simulink model "AFE_3L_DCP_DCN"  (R2013a)
settings: Solver=FixedStepDiscrete  SolverMode=SingleTasking  StartTime=0.0  StopTime=inf  FixedStep=Tpas  RelTol=1e-3
values from neighbouring files (symbols this model uses):
  Cbus = 300e-3    (= 0.3)    [AFE_FV_Params.m]
  fmod4Q = 1e3    (= 1000)    [AFE_FV_Params.m]
  Freq = 50    [AFE_FV_Params.m]
  IC = 2    [AFE_FV_Params.m]
  IDCP = (PDCP+Numd(2)/Dend(1))/Ts    [AFE_FV_Params.m]
  Iv = (Pv+Numdv(2)/Dendv(1))/Tsv    [AFE_FV_Params.m]
  Kac = 1/(Vac*sqrt(2/3))    [AFE_FV_Params.m]
  L = .1    (= 0.1)    [AFE_FV_Params.m]
  Lac = 8.1487e-04    (= 0.00081487)    [AFE_FV_Params.m]
  Lcoup = 10e-6    (= 1e-05)    [AFE_FV_Params.m]
  PC = 0.001    [AFE_FV_Params.m]
  PDCP = Numd(1)/Dend(1)    [AFE_FV_Params.m]
  Pv = Numdv(1)/Dendv(1)    [AFE_FV_Params.m]
  R = .28    (= 0.28)    [AFE_FV_Params.m]
  Satv = 1000    [AFE_FV_Params.m]
  Tpas = 1e-6    (= 1e-06)    [AFE_FV_Params.m]
  Vac = 2000    [AFE_FV_Params.m]
  Vdc = 5000    [AFE_FV_Params.m]
undefined symbols (not defined in the file or in its folder): KLPDCP, Rac, TLPDCP
libraries: powerlib x78, simulink x46, powerlib_meascontrol x16
settings Model: Creator=LiberT  LastModifiedBy=Francis
settings DataIOCC: SignalLoggingSaveFormat=ModelDataLogs
settings OptimizationCC: ExpressionDepthLimit=2147483647
settings DebuggingCC: MultiTaskDSMMsg=warning  MultiTaskCondExecSysMsg=none  FcnCallInpInsideContextMsg=EnableAllAsWarning  StrictBusMsg=None
settings RTWCC: IncludeERTFirstTime=on

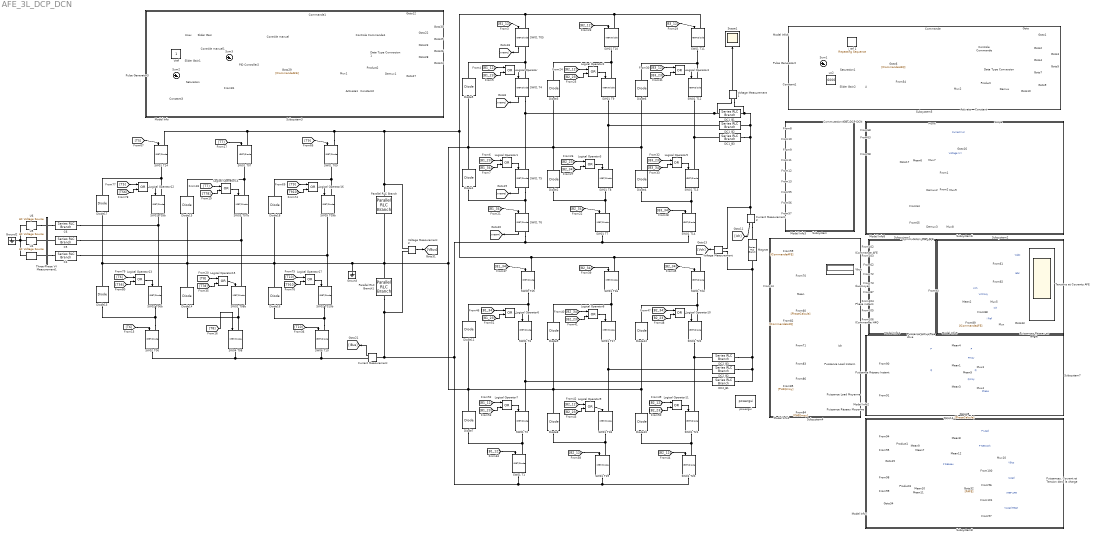
== system AFE_3L_DCP_DCN ==
  " " : ManualSwitch
  " 4" : ManualSwitch  CurrentSetting=0
  Activate : Constant  Value=0
  Activate1 : Constant  Value=0
  C4 : powerlib/Elements/Series RLC Branch  LConnTagsString=__new0  RConnTagsString=__new0  BranchType=L  Resistance=Rac  Inductance=Lac  SetiL0=off  InitialCurrent=0  Capacitance=300e-3  Setx0=off  InitialVoltage=0  Measurements=None
  C5 : powerlib/Elements/Series RLC Branch  LConnTagsString=__new0  RConnTagsString=__new0  BranchType=L  Resistance=Rac  Inductance=Lac  SetiL0=off  InitialCurrent=0  Capacitance=300e-3  Setx0=off  InitialVoltage=0  Measurements=None
  C6 : powerlib/Elements/Series RLC Branch  LConnTagsString=__new0  RConnTagsString=__new0  BranchType=L  Resistance=Rac  Inductance=Lac  SetiL0=off  InitialCurrent=0  Capacitance=300e-3  Setx0=off  InitialVoltage=0  Measurements=None
  Commande : Subsystem
  Commande1 : Subsystem
  Commutation IGBT AFE : Scope  NumInputPorts=9
      settings: TickLabels=on  TimeRange=0.04  YMin=-0.2~-0.2~-0.2~-0.2~-0.2~-0.2~-5~-5~-5  YMax=1.2~1.2~1.2~1.2~1.2~1.2~5~5~5  SaveName=ScopeData4
  Commutation IGBT DCP-DCN : Scope  NumInputPorts=9
      settings: TickLabels=on  TimeRange=0.04  YMin=-0.2~-0.2~-0.2~-0.2~-0.2~-0.2~-0.2~-0.2~-0.2  YMax=1.2~1.2~1.2~1.2~1.2~1.2~1.2~1.2~1.2
  Constant : Constant  Value=[1 1 1 1 1 1 1 1 1]
  Constant1 : Constant  Value=6000
  Constant2 : Constant  Value=[1 1 1 1 1 1 1 1 1]
  Constant3 : Constant  Value=6000
  Controle Commande : ManualSwitch
  Controle Commande1 : ManualSwitch
  Contrôle manuel : ManualSwitch  CurrentSetting=0
  Contrôle manuel1 : ManualSwitch
  Current Measurement : powerlib/Measurements/Current Measurement  PhasorSimulation=off  OutputType=Complex  PSBequivalent=0
  Current Measurement2 : powerlib/Measurements/Current Measurement  PhasorSimulation=off  OutputType=Complex  PSBequivalent=0
  DC1_B1 : powerlib/Elements/Series RLC Branch  LConnTagsString=__new0  RConnTagsString=__new0  BranchType=L  Resistance=0  Inductance=Lcoup  SetiL0=off  InitialCurrent=0  Capacitance=1e-6  Setx0=off  InitialVoltage=0  Measurements=Branch current
  DC1_B2 : powerlib/Elements/Series RLC Branch  LConnTagsString=__new0  RConnTagsString=__new0  BranchType=L  Resistance=0  Inductance=Lcoup  SetiL0=off  InitialCurrent=0  Capacitance=1e-6  Setx0=off  InitialVoltage=0  Measurements=Branch current
  DC1_B3 : powerlib/Elements/Series RLC Branch  LConnTagsString=__new0  RConnTagsString=__new0  BranchType=L  Resistance=0  Inductance=Lcoup  SetiL0=off  InitialCurrent=0  Capacitance=1e-6  Setx0=off  InitialVoltage=0  Measurements=Branch current
  "DC2_B1 " : powerlib/Elements/Series RLC Branch  LConnTagsString=__new0  RConnTagsString=__new0  BranchType=L  Resistance=0  Inductance=Lcoup  SetiL0=off  InitialCurrent=0  Capacitance=1e-6  Setx0=off  InitialVoltage=0  Measurements=Branch current
  DC2_B2 : powerlib/Elements/Series RLC Branch  LConnTagsString=__new0  RConnTagsString=__new0  BranchType=L  Resistance=0  Inductance=Lcoup  SetiL0=off  InitialCurrent=0  Capacitance=1e-6  Setx0=off  InitialVoltage=0  Measurements=Branch current
  DC2_B3 : powerlib/Elements/Series RLC Branch  LConnTagsString=__new0  RConnTagsString=__new0  BranchType=L  Resistance=0  Inductance=Lcoup  SetiL0=off  InitialCurrent=0  Capacitance=1e-6  Setx0=off  InitialVoltage=0  Measurements=Branch current
  Data Type Conversion : DataTypeConversion  OutDataTypeStr=boolean
  Data Type Conversion1 : DataTypeConversion  OutDataTypeStr=boolean
  Demux : Demux  Outputs=9
  Demux1 : Demux  Outputs=9
  Demux2 : Demux  Outputs=2
  Demux3 : Demux  Outputs=2
  Diode{1..18} (18 alike) : powerlib/Power Electronics/Diode  Ron=0.001  Lon=0  Vf=0.8  IC=0  UseSnubber=off  Rs=500  Cs=inf  Measurements=off
  Ground : powerlib/Elements/Ground  LConnTagsString=a
  Ground2 : powerlib/Elements/Ground  LConnTagsString=a
  "ICommande AFE " : Display
  ICommande H4Q : Display
  Ibusmoyen : Display
  Ich : Display
  Imax : Constant  Value=5000
  Logical Operator{,1..17} (18 alike) : Logic  Operator=OR  AllPortsSameDT=off  OutDataTypeStr=boolean
  Magnet : powerlib/Elements/Series RLC Branch  LConnTagsString=__new0  RConnTagsString=__new0  BranchType=RL  Resistance=R  Inductance=L  SetiL0=off  InitialCurrent=0  Capacitance=1e-6  Setx0=off  InitialVoltage=0  Measurements=Branch voltage and current
  Mean{,1..3} (4 alike) : powerlib_meascontrol/Measurements/Mean  Freq=50  Vinit=0  Ts=Tpas
  Mean10 : powerlib_meascontrol/Measurements/Mean  Freq=fmod4Q/2  Vinit=0  Ts=Tpas
  Mean11 : powerlib_meascontrol/Measurements/Mean  Freq=1/.9  Vinit=0  Ts=Tpas
  Mean12 : powerlib_meascontrol/Measurements/Mean  Freq=fmod4Q  Vinit=0  Ts=Tpas
  Mean4 : powerlib_meascontrol/Measurements/Mean  Freq=fmod4Q*3  Vinit=0  Ts=Tpas
  Mean5 : powerlib_meascontrol/Measurements/Mean  Freq=fmod4Q*3  Vinit=0  Ts=Tpas
  Mean6 : powerlib_meascontrol/Measurements/Mean  Freq=fmod4Q/3  Vinit=0  Ts=Tpas
  Mean7 : powerlib_meascontrol/Measurements/Mean  Freq=1/.9  Vinit=0  Ts=Tpas
  Mean8 : powerlib_meascontrol/Measurements/Mean  Freq=fmod4Q  Vinit=0  Ts=Tpas
  Mean9 : powerlib_meascontrol/Measurements/Mean  Freq=fmod4Q/2  Vinit=0  Ts=Tpas
  Model Info : simulink/Model-Wide Utilities/Model Info  InitialBlockCM=None  BlockCM=None  Frame=on  DisplayStringWithTags=Commande AFE  HorizontalTextAlignment=Center  LeftAlignmentValue=0.5  SourceBlockDiagram=AFE_3L_DCP_DCN  TagMaxNumber=20
  Model Info{1..5,7..8} (7 alike) : simulink/Model-Wide Utilities/Model Info  InitialBlockCM=None  BlockCM=None  Frame=on  DisplayStringWithTags=Résultats  HorizontalTextAlignment=Center  LeftAlignmentValue=0.5  SourceBlockDiagram=AFE_3L_DCP_DCN  TagMaxNumber=20
  Model Info6 : simulink/Model-Wide Utilities/Model Info  InitialBlockCM=None  BlockCM=None  Frame=on  DisplayStringWithTags=Commande H4Q  HorizontalTextAlignment=Center  LeftAlignmentValue=0.5  SourceBlockDiagram=AFE_3L_DCP_DCN  TagMaxNumber=20
  Mux{,3..10} (9 alike) : Mux  Inputs=2
  Mux1 : Mux  Inputs=9
  Mux2 : Mux  Inputs=9
  PID Controller2 : simulink/Continuous/PID Controller  Controller=PI  TimeDomain=Discrete-time  SampleTime=Tpas  IntegratorMethod=Forward Euler  FilterMethod=Forward Euler  Form=Parallel  P=Pv  I=Iv  D=0  N=100  InitialConditionSource=internal  InitialConditionForIntegrator=0  InitialConditionForFilter=0  ExternalReset=none  LimitOutput=on  UpperSaturationLimit=Satv  LowerSaturationLimit=-Satv  LinearizeAsGain=on  AntiWindupMode=clamping  Kb=1  TrackingMode=off  Kt=1  PParamMin=[]  PParamMax=[]  IParamMin=[]  IParamMax=[]  DParamMin=[]  DParamMax=[]  NParamMin=[]  NParamMax=[]  KbParamMin=[]  KbParamMax=[]  KtParamMin=[]  KtParamMax=[]  POutMin=[]  POutMax=[]  IOutMin=[]  IOutMax=[]  DOutMin=[]  DOutMax=[]  NOutMin=[]  NOutMax=[]  KbOutMin=[]  KbOutMax=[]  KtOutMin=[]  KtOutMax=[]  IntegratorOutMin=[]  IntegratorOutMax=[]  FilterOutMin=[]  FilterOutMax=[]  SumOutMin=[]  SumOutMax=[]  SumI1OutMin=[]  SumI1OutMax=[]  SumI2OutMin=[]  SumI2OutMax=[]  SumI3OutMin=[]  SumI3OutMax=[]  SumDOutMin=[]  SumDOutMax=[]  SaturationOutMin=[]  SaturationOutMax=[]  IntegratorContinuousStateAttributes=''  IntegratorStateMustResolveToSignalObject=off  IntegratorRTWStateStorageClass=Auto  FilterContinuousStateAttributes=''  FilterStateMustResolveToSignalObject=off  FilterRTWStateStorageClass=Auto
  Parallel RLC Branch : powerlib/Elements/Parallel RLC Branch  LConnTagsString=a  RConnTagsString=__new0  BranchType=C  Resistance=9.26  Inductance=1e-3  SetiL0=off  InitialCurrent=0  Capacitance=Cbus*2  Setx0=on  InitialVoltage=Vdc/2  Measurements=None
  Parallel RLC Branch1 : powerlib/Elements/Parallel RLC Branch  LConnTagsString=a  RConnTagsString=__new0  BranchType=C  Resistance=9.26  Inductance=1e-3  SetiL0=off  InitialCurrent=0  Capacitance=Cbus*2  Setx0=on  InitialVoltage=Vdc/2  Measurements=None
  Phase instant. : Display
  Product{,1..3} (4 alike) : Product
  Puissance Active/Reactive : Subsystem
  Puissance Load Instant. : Display
  Puissance Load Moyenne : Display
  Puissance Réseau Instant : Display
  Puissance Réseau Moyenne : Display
  Puissances Réseau et angle : Scope  NumInputPorts=3
      settings: TickLabels=on  TimeRange=0.04  YMin=-1000000~-400000~-200  YMax=10000000~350000~200  SaveName=ScopeData2
  "Puissances, Courant et Tension dans la charge" : Scope  NumInputPorts=5
      settings: TickLabels=on  ShowLegends=on  TimeRange=0.9  YMin=-20000000~3000~-1000~-3000~-5000  YMax=20000000~8000~7000~3000~5000  SaveName=ScopeData7
  Pulse Generator2 : DiscretePulseGenerator  Amplitude=12000  Period=floor(.4 /Tpas)  PulseWidth=floor(.4 * .5 / Tpas)  PhaseDelay=floor(.001 / Tpas)  SampleTime=Tpas
  Pulse Generator3 : DiscretePulseGenerator  Amplitude=12000  Period=floor(.2/Tpas)  PulseWidth=floor(.2/2/Tpas)  SampleTime=Tpas
  SW01 T05 : powerlib/Power Electronics/IGBT//Diode  Ron=Ron  Rs=Rs  Cs=Cs  Measurements=on
  SW01 T05b : powerlib/Power Electronics/IGBT//Diode  Ron=1e-3  Rs=1e5  Cs=Tpas  Measurements=off
  SW01 T07 : powerlib/Power Electronics/IGBT//Diode  Ron=1e-3  Rs=1e5  Cs=Tpas  Measurements=off
  SW01 T09 : powerlib/Power Electronics/IGBT//Diode  Ron=1e-3  Rs=1e5  Cs=Tpas  Measurements=off
  SW01 T{1..3,7..23} (20 alike) : powerlib/Power Electronics/IGBT//Diode  Ron=Ron  Rs=Rs  Cs=Cs  Measurements=off
  SW01 T24 : powerlib/Power Electronics/IGBT//Diode  Ron=1e-3  Rs=1e5  Cs=Tpas  Measurements=off
  SW01 T4 : powerlib/Power Electronics/IGBT//Diode  Ron=Ron  Rs=Rs  Cs=Cs  Measurements=on
  SW01 T5 : powerlib/Power Electronics/IGBT//Diode  Ron=Ron  Rs=Rs  Cs=Cs  Measurements=on
  SW01 T6 : powerlib/Power Electronics/IGBT//Diode  Ron=Ron  Rs=Rs  Cs=Cs  Measurements=on
  SW02 T010b : powerlib/Power Electronics/IGBT//Diode  Ron=1e-3  Rs=1e5  Cs=Tpas  Measurements=off
  SW02 T06 : powerlib/Power Electronics/IGBT//Diode  Ron=1e-3  Rs=1e5  Cs=Tpas  Measurements=off
  SW02 T06b : powerlib/Power Electronics/IGBT//Diode  Ron=1e-3  Rs=1e5  Cs=Tpas  Measurements=off
  SW02 T08b : powerlib/Power Electronics/IGBT//Diode  Ron=1e-3  Rs=1e5  Cs=Tpas  Measurements=off
  SW03 T07b : powerlib/Power Electronics/IGBT//Diode  Ron=1e-3  Rs=1e5  Cs=Tpas  Measurements=off
  SW04 T08 : powerlib/Power Electronics/IGBT//Diode  Ron=1e-3  Rs=1e5  Cs=Tpas  Measurements=off
  SW05 T09b : powerlib/Power Electronics/IGBT//Diode  Ron=1e-3  Rs=1e5  Cs=Tpas  Measurements=off
  SW06 T10 : powerlib/Power Electronics/IGBT//Diode  Ron=1e-3  Rs=1e5  Cs=Tpas  Measurements=off
  Saturation : Saturate  UpperLimit=5100  LowerLimit=5000
  Saturation1 : Saturate  UpperLimit=5000  LowerLimit=2000
  Scope : Scope  NumInputPorts=6
      settings: TimeRange=0.9  YMin=-7000~-5000~-0.1~-0.1~-15000~0  YMax=7000~5000~1.1~1.1~15000~2500  SaveName=ScopeData5  MaxDataPoints=10000
  Scope1 : Scope
      settings: TimeRange=0.9  YMin=-7000  YMax=7000  SaveName=ScopeData6  MaxDataPoints=10000
  Slider Gain : simulink/Math Operations/Slider Gain  low=0  gain=0.22  high=1
  Slider Gain1 : simulink/Math Operations/Slider Gain  low=0  gain=5000  high=6000
  Slider Gain2 : simulink/Math Operations/Slider Gain  low=0  gain=0.54  high=1
  Subsystem : Subsystem
      mask Display: disp('')
  Subsystem1 : Subsystem
      mask Display: disp('')
  Subsystem2 : Subsystem
      mask Display: disp('')
  Subsystem3 : Subsystem
      mask Display: disp('')
  Subsystem4 : Subsystem
      mask Display: disp('')
  Subsystem5 : Subsystem
      mask Display: disp('')
  Subsystem6 : Subsystem
      mask Display: disp('')
  Subsystem7 : Subsystem
      mask Display: disp('')
  Subsystem8 : Subsystem
      mask Display: disp('')
  Sum1 : Sum  Inputs=|+-
  Sum2 : Sum  Inputs=|+-
  Sum3 : Sum  Inputs=|+-
  Tensions et Courants AFE : Scope  NumInputPorts=4
      settings: TickLabels=on  ShowLegends=on  TimeRange=0.04  YMin=-1750~-2000~3000~-2000  YMax=1750~2000~5150~2000
  Three-Phase V-I Measurement1 : powerlib/Measurements/Three-Phase V-I Measurement  VoltageMeasurement=phase-to-ground  SetLabelV=on  LabelV=Vabc  Vpu=off  VpuLL=off  CurrentMeasurement=yes  SetLabelI=on  LabelI=Iabc  Ipu=off  Pbase=100e6  Vbase=500e3  OutputType=Complex  PhasorSimulation=off  PSBequivalent=0
  U4 : powerlib/Electrical Sources/AC Voltage Source  Amplitude=Vac*sqrt(2/3)  Phase=120  Frequency=Freq  SampleTime=Tpas  Measurements=Voltage
  U5 : powerlib/Electrical Sources/AC Voltage Source  Amplitude=Vac*sqrt(2/3)  Phase=-120  Frequency=Freq  SampleTime=Tpas  Measurements=Voltage
  U6 : powerlib/Electrical Sources/AC Voltage Source  Amplitude=Vac*sqrt(2/3)  Phase=0  Frequency=Freq  SampleTime=Tpas  Measurements=Voltage
  Vbus : Display
  Voltage Measurement : powerlib/Measurements/Voltage Measurement  PhasorSimulation=off  OutputType=Complex  PSBequivalent=0
  Voltage Measurement1 : powerlib/Measurements/Voltage Measurement  PhasorSimulation=off  OutputType=Complex  PSBequivalent=0
  Voltage Measurement2 : powerlib/Measurements/Voltage Measurement  PhasorSimulation=off  OutputType=Complex  PSBequivalent=0
  Vref : Constant  SampleTime=Tpas
  i_ref 1 : simulink/Sources/Repeating Sequence  rep_seq_t="[0 108.51e-3 127.6e-3 132e-3 200e-3 250e-3 283.33e-3 310e-3 366.66e-3  490e-3 533e-3 683.33e-3 900e-3]"  rep_seq_y=[333 333 1000 1031 1500 2000 2500 3000 4000 6000 6000 333 333]
  powergui : powerlib/powergui  Priority=1  SimulationMode=Discrete  SolverType=Tustin  SampleTime=Tpas  frequency=60  SPID=off  DisableSnubberDevices=off  DisableRonSwitches=off  DisableVfSwitches=off  SwTol=0  Interpol=off  DisplayEquations=off  frequencyindice=50  Pbase=100e6  ErrMax=1e-4  Iterations=50  UnitsV=kV  UnitsW=MW  FunctionMessages=off  echomessages=off  HookPort=off  EnableUseOfTLC=off  x0status=blocks  RestoreLinks=warning  ResistiveCurrentMeasurement=off  Frange=[0:2:500]  Ylog=off  Xlog=on  ShowGrid=off  save=off  variable=ZData  structure=ScopeData1  ZoomFFT=off  StartTime=18  cycles=100  DisplayStyle=1  fundamental=50  FreqAxis=off  MaxFrequency=2000  frequencyindicesteady=1  RmsSteady=1  display=off  Ts=0  methode=off
  uo2 : Constant  Value=6000
  wires:
  [B1_12] -> Commutation IGBT DCP-DCN/1
  [B1_23] -> Commutation IGBT DCP-DCN/2
  [B1_34] -> Commutation IGBT DCP-DCN/3
  [B2_12] -> Commutation IGBT DCP-DCN/4
  [B2_23] -> Commutation IGBT DCP-DCN/5
  [B2_34] -> Commutation IGBT DCP-DCN/6
  Constant/1 -> Product/2
  Activate/1 -> Product/1
  Controle Commande/1 -> Demux/1
  Mux2/1 -> Controle Commande/1
  Data Type Conversion/1 -> Controle Commande/2
  Product/1 -> Data Type Conversion/1
  Commande/1(12_B1) -> Mux2/1
  Commande/2(23_B1) -> Mux2/2
  Commande/3(34_B1) -> Mux2/3
  Demux/1 -> [B1_12]
  Demux/3 -> [B1_34]
  Demux/2 -> [B1_23]
  [B1_12] -> SW01 T05/1
  Logical Operator/1 -> SW01 T4/1
  [B1_12] -> Logical Operator/1
  [B1_23] -> Logical Operator/2
  Logical Operator1/1 -> SW01 T5/1
  [B1_23] -> Logical Operator1/1
  [B1_34] -> Logical Operator1/2
  [B1_34] -> SW01 T6/1
  [B2_12] -> SW01 T10/1
  Logical Operator2/1 -> SW01 T9/1
  [B2_12] -> Logical Operator2/1
  [B2_23] -> Logical Operator2/2
  Logical Operator3/1 -> SW01 T8/1
  [B2_23] -> Logical Operator3/1
  [B2_34] -> Logical Operator3/2
  [B2_34] -> SW01 T7/1
  [B3_12] -> SW01 T11/1
  Logical Operator4/1 -> SW01 T12/1
  [B3_12] -> Logical Operator4/1
  [B3_23] -> Logical Operator4/2
  Logical Operator5/1 -> SW01 T13/1
  [B3_23] -> Logical Operator5/1
  [B3_34] -> Logical Operator5/2
  [B3_34] -> SW01 T14/1
  [B1_34] -> SW01 T15/1
  Logical Operator6/1 -> SW01 T3/1
  [B1_34] -> Logical Operator6/1
  [B1_23] -> Logical Operator6/2
  Logical Operator7/1 -> SW01 T2/1
  [B1_12] -> Logical Operator7/1
  [B1_23] -> Logical Operator7/2
  [B1_12] -> SW01 T1/1
  [B2_34] -> SW01 T16/1
  Logical Operator8/1 -> SW01 T17/1
  [B2_34] -> Logical Operator8/1
  [B2_23] -> Logical Operator8/2
  Logical Operator9/1 -> SW01 T18/1
  [B2_12] -> Logical Operator9/1
  [B2_23] -> Logical Operator9/2
  [B2_12] -> SW01 T19/1
  [B2_34] -> SW01 T23/1
  Logical Operator10/1 -> SW01 T22/1
  [B2_34] -> Logical Operator10/1
  [B2_23] -> Logical Operator10/2
  Logical Operator11/1 -> SW01 T21/1
  [B2_12] -> Logical Operator11/1
  [B2_23] -> Logical Operator11/2
  [B2_12] -> SW01 T20/1
  uo2/1 -> Slider Gain2/1
  Slider Gain2/1 -> " 4"/2
  Saturation1/1 -> " 4"/1
  Constant1/1 -> Sum1/2
  i_ref 1/1 -> " "/1
  " 4"/1 -> " "/2
  Pulse Generator2/1 -> Sum1/1
  Sum1/1 -> Saturation1/1
  " "/1 -> Commande/1(Iref), [ICommandeH4Q]
  Commande/4(12_B2) -> Mux2/4
  Commande/5(23_B2) -> Mux2/5
  Commande/6(34_B2) -> Mux2/6
  Commande/7(12_B3) -> Mux2/7
  Commande/8(23_B3) -> Mux2/8
  Commande/9(34_B3) -> Mux2/9
  Demux/4 -> [B2_12]
  Demux/6 -> [B2_34]
  Demux/5 -> [B2_23]
  Demux/7 -> [B3_12]
  Demux/9 -> [B3_34]
  Demux/8 -> [B3_23]
  Current Measurement2/1 -> [Ich]
  Voltage Measurement/1 -> [Vch]
  [Ich] -> Commande/2("Iload ")
  [B3_12] -> Commutation IGBT DCP-DCN/7
  [B3_23] -> Commutation IGBT DCP-DCN/8
  [B3_34] -> Commutation IGBT DCP-DCN/9
  Mux6/1 -> [ILoadScope], Scope/1  "Current (A)"
  Mux7/1 -> Scope/2  "Voltage (V)"
  [Ich] -> Mux6/2
  [mIGBT1] -> Demux2/1
  Mean6/1 -> [VMeanLoad], Mux7/2
  [Vch] -> Mux7/1, Mean6/1
  [mIGBT2] -> Demux3/1
  [B1_12] -> Scope/3
  Mux8/1 -> Scope/6
  Mux9/1 -> Scope/5
  [B1_34] -> Scope/4
  Demux2/1 -> Mux9/1
  Demux3/1 -> Mux9/2
  Demux2/2 -> Mux8/1
  Demux3/2 -> Mux8/2
  [ICommandeH4Q] -> Mux6/1
  SW01 T4/1 -> [mIGBT2]
  SW01 T05/1 -> [mIGBT1]
  SW01 T5/1 -> [mIGBT3]
  SW01 T6/1 -> [mIGBT4]
  Voltage Measurement1/1 -> Scope1/1
  Current Measurement/1 -> [IBus]
  [T5] -> SW01 T24/1
  Logical Operator12/1 -> SW01 T05b/1
  [T5] -> Logical Operator12/1
  [T56] -> Logical Operator12/2
  Logical Operator13/1 -> SW02 T06b/1
  [T6] -> Logical Operator13/1
  [T56] -> Logical Operator13/2
  [T6] -> SW02 T06/1
  [T7] -> SW01 T07/1
  Logical Operator14/1 -> SW03 T07b/1
  [T7] -> Logical Operator14/1
  [T78] -> Logical Operator14/2
  Logical Operator15/1 -> SW02 T08b/1
  [T8] -> Logical Operator15/1
  [T78] -> Logical Operator15/2
  [T8] -> SW04 T08/1
  [T9] -> SW01 T09/1
  Logical Operator16/1 -> SW05 T09b/1
  [T9] -> Logical Operator16/1
  [T910] -> Logical Operator16/2
  Logical Operator17/1 -> SW02 T010b/1
  [T10] -> Logical Operator17/1
  [T910] -> Logical Operator17/2
  [T10] -> SW06 T10/1
  Imax/1 -> Slider Gain/1
  [VBus] -> Sum3/2
  Vref/1 -> Slider Gain1/1
  Sum3/1 -> PID Controller2/1
  Constant2/1 -> Product2/2
  Activate1/1 -> Product2/1
  Controle Commande1/1 -> Demux1/1
  Mux1/1 -> Controle Commande1/1
  PID Controller2/1 -> Contrôle manuel/2
  Slider Gain/1 -> Contrôle manuel/1
  Contrôle manuel/1 -> [ICommandeAFE], Commande1/1(In1)
  Data Type Conversion1/1 -> Controle Commande1/2
  Product2/1 -> Data Type Conversion1/1
  Sum2/1 -> Saturation/1
  Pulse Generator3/1 -> Sum2/1
  Constant3/1 -> Sum2/2
  Contrôle manuel1/1 -> Sum3/1
  Slider Gain1/1 -> Contrôle manuel1/1
  Saturation/1 -> Contrôle manuel1/2
  Commande1/1(T5) -> Mux1/1
  Commande1/2(T56) -> Mux1/2
  Commande1/3(T6) -> Mux1/3
  Commande1/4(T7) -> Mux1/4
  Commande1/5(T78) -> Mux1/5
  Commande1/6(T8) -> Mux1/6
  Commande1/7(T9) -> Mux1/7
  Commande1/8(T89) -> Mux1/8
  Commande1/9(T10) -> Mux1/9
  Demux1/1 -> [T5]
  Demux1/3 -> [T6]
  Demux1/4 -> [T7]
  Demux1/6 -> [T8]
  Demux1/7 -> [T9]
  Demux1/9 -> [T10]
  Demux1/2 -> [T56]
  Demux1/5 -> [T78]
  Demux1/8 -> [T910]
  Voltage Measurement2/1 -> [VBus]
  Mean/1 -> Ibusmoyen/1
  [VBus] -> Vbus/1
  [IBus] -> Mean/1
  [ICommandeAFE] -> "ICommande AFE "/1
  [PhaseCalcule] -> Phase instant./1
  [PAFEmoy] -> Puissance Réseau Moyenne/1
  [PH4Q] -> Puissance Load Instant./1
  [Ich] -> Ich/1
  [ICommandeH4Q] -> ICommande H4Q/1
  [PAFE] -> Puissance Réseau Instant/1
  [PH4Qmoy] -> Puissance Load Moyenne/1
  [T5] -> Commutation IGBT AFE/1
  [T56] -> Commutation IGBT AFE/2
  [T6] -> Commutation IGBT AFE/3
  [T7] -> Commutation IGBT AFE/4
  [T78] -> Commutation IGBT AFE/5
  [T8] -> Commutation IGBT AFE/6
  [Vabc] -> Tensions et Courants AFE/1  "Vabc"
  [Iabc] -> Tensions et Courants AFE/2  "Iabc"
  [IBus] -> Mux/1  "Ich"
  [ICommandeAFE] -> Mux/2  "I Ref"
  Mux/1 -> [IBusScope], Tensions et Courants AFE/4
  [Vabc] -> Puissance Active/Reactive/1(Vabc)
  [Iabc] -> Puissance Active/Reactive/2(Iabc)
  Puissance Active/Reactive/1(P) -> Mean4/1, Mean1/1  "P"
  Puissance Active/Reactive/2(Q) -> Mean3/1, Mean5/1  "Q"
  Puissance Active/Reactive/3(PhC) -> Puissances Réseau et angle/3, [PhaseCalcule]  "Phase"
  Mean1/1 -> Mux3/2  "Pmoy"
  Mux3/1 -> Puissances Réseau et angle/1
  Mean3/1 -> Mux4/2  "Qmoy"
  Mux4/1 -> Puissances Réseau et angle/2
  Mux5/1 -> Tensions et Courants AFE/3
  [VBus] -> Mux5/1, Mean2/1  "Vch"
  Mean2/1 -> Mux5/2  "Vchmoy"
  Mean4/1 -> Mux3/1  "P"
  Mean5/1 -> Mux4/1  "Q"
  Mean7/1 -> [PH4Qmoy]
  [Vch] -> Product1/1
  [Ich] -> Product1/2
  Product1/1 -> Mean9/1
  Mean9/1 -> Mean7/1, Mean8/1
  Mean8/1 -> [PH4Q], Mux10/1  "P Load"
  [VMeanLoad] -> "Puissances, Courant et Tension dans la charge"/5  "VLoad Mean"
  Mux10/1 -> "Puissances, Courant et Tension dans la charge"/1
  [VBus] -> "Puissances, Courant et Tension dans la charge"/2  "VBus"
  [ILoadScope] -> "Puissances, Courant et Tension dans la charge"/3  "ILoad"
  [ICommandeAFE] -> "Puissances, Courant et Tension dans la charge"/4  "I REF AFE"
  [IBus] -> Product3/1
  [VBus] -> Product3/2
  Product3/1 -> Mean10/1
  Mean10/1 -> Mean11/1, Mean12/1  "P Réseau"
  Mean11/1 -> [PAFEmoy]
  Mean12/1 -> [PAFE], Mux10/2  "P Network"
  [T9] -> Commutation IGBT AFE/7
  [T910] -> Commutation IGBT AFE/8
  [T100] -> Commutation IGBT AFE/9
  connections:
  DC1_B1/LConn1 -- SW01 T5/LConn1 -- SW01 T4/RConn1 -- Voltage Measurement1/LConn1
  DC1_B3/LConn1 -- SW01 T13/LConn1 -- SW01 T12/RConn1
  DC1_B2/LConn1 -- SW01 T9/RConn1 -- SW01 T8/LConn1
  Diode5/RConn1 -- SW01 T05/RConn1 -- SW01 T4/LConn1
  Diode3/RConn1 -- SW01 T10/RConn1 -- SW01 T9/LConn1
  Diode6/RConn1 -- SW01 T12/LConn1 -- SW01 T11/RConn1
  Diode1/LConn1 -- SW01 T6/LConn1 -- SW01 T5/RConn1
  Diode4/LConn1 -- SW01 T14/LConn1 -- SW01 T13/RConn1
  Diode2/LConn1 -- SW01 T8/RConn1 -- SW01 T7/LConn1
  Parallel RLC Branch1/RConn1 -- Voltage Measurement2/LConn2 -- Current Measurement/LConn1 -- SW01 T1/RConn1 -- SW01 T20/RConn1 -- SW01 T19/RConn1 -- SW01 T6/RConn1 -- SW01 T14/RConn1 -- SW01 T7/RConn1
  SW01 T09/LConn1 -- Voltage Measurement2/LConn1 -- Parallel RLC Branch/LConn1 -- SW01 T11/LConn1 -- SW01 T10/LConn1 -- SW01 T05/LConn1 -- SW01 T23/LConn1 -- SW01 T16/LConn1 -- SW01 T15/LConn1 -- SW01 T24/LConn1 -- SW01 T07/LConn1
  Diode11/RConn1 -- SW01 T15/RConn1 -- SW01 T3/LConn1
  Diode9/RConn1 -- SW01 T17/LConn1 -- SW01 T16/RConn1
  Diode12/RConn1 -- SW01 T23/RConn1 -- SW01 T22/LConn1
  Diode7/LConn1 -- SW01 T2/RConn1 -- SW01 T1/LConn1
  Diode10/LConn1 -- SW01 T21/RConn1 -- SW01 T20/LConn1
  Diode8/LConn1 -- SW01 T19/LConn1 -- SW01 T18/RConn1
  Diode13/RConn1 -- Diode17/LConn1 -- Diode15/LConn1 -- Diode14/RConn1 -- Diode16/RConn1 -- Diode18/LConn1 -- Ground/LConn1 -- Parallel RLC Branch1/LConn1 -- Diode11/LConn1 -- Diode7/RConn1 -- Diode9/LConn1 -- Diode8/RConn1 -- Diode10/RConn1 -- Diode12/LConn1 -- Diode4/RConn1 -- Diode6/LConn1 -- Diode3/LConn1 -- Diode2/RConn1 -- Diode5/LConn1 -- Diode1/RConn1 -- Parallel RLC Branch/RConn1
  SW01 T21/LConn1 -- DC2_B3/RConn1 -- SW01 T22/RConn1
  SW01 T2/LConn1 -- "DC2_B1 "/RConn1 -- SW01 T3/RConn1
  SW01 T17/RConn1 -- DC2_B2/RConn1 -- SW01 T18/LConn1
  DC1_B1/RConn1 -- Voltage Measurement/LConn1 -- Current Measurement2/LConn1 -- DC1_B3/RConn1 -- DC1_B2/RConn1 -- Voltage Measurement1/LConn2
  DC2_B3/LConn1 -- "DC2_B1 "/LConn1 -- DC2_B2/LConn1 -- Voltage Measurement/LConn2 -- Magnet/RConn1
  Current Measurement2/RConn1 -- Magnet/LConn1
  C6/LConn1 -- SW02 T06b/LConn1 -- SW01 T05b/RConn1
  SW05 T09b/RConn1 -- SW02 T010b/LConn1 -- C4/LConn1
  SW03 T07b/RConn1 -- SW02 T08b/LConn1 -- C5/LConn1
  SW01 T24/RConn1 -- SW01 T05b/LConn1 -- Diode17/RConn1
  SW01 T07/RConn1 -- SW03 T07b/LConn1 -- Diode15/RConn1
  SW01 T09/RConn1 -- SW05 T09b/LConn1 -- Diode18/RConn1
  SW02 T06/LConn1 -- SW02 T06b/RConn1 -- Diode13/LConn1
  SW06 T10/LConn1 -- SW02 T010b/RConn1 -- Diode16/LConn1
  SW02 T08b/RConn1 -- SW04 T08/LConn1 -- Diode14/LConn1
  SW04 T08/RConn1 -- SW02 T06/RConn1 -- SW06 T10/RConn1 -- Current Measurement/RConn1
  U5/LConn1 -- Ground2/LConn1 -- U4/LConn1 -- U6/LConn1
  Three-Phase V-I Measurement1/RConn3 -- U4/RConn1
  Three-Phase V-I Measurement1/RConn2 -- U5/RConn1
  Three-Phase V-I Measurement1/LConn1 -- C6/RConn1
  C5/RConn1 -- Three-Phase V-I Measurement1/LConn2
  U6/RConn1 -- Three-Phase V-I Measurement1/RConn1
  Three-Phase V-I Measurement1/LConn3 -- C4/RConn1

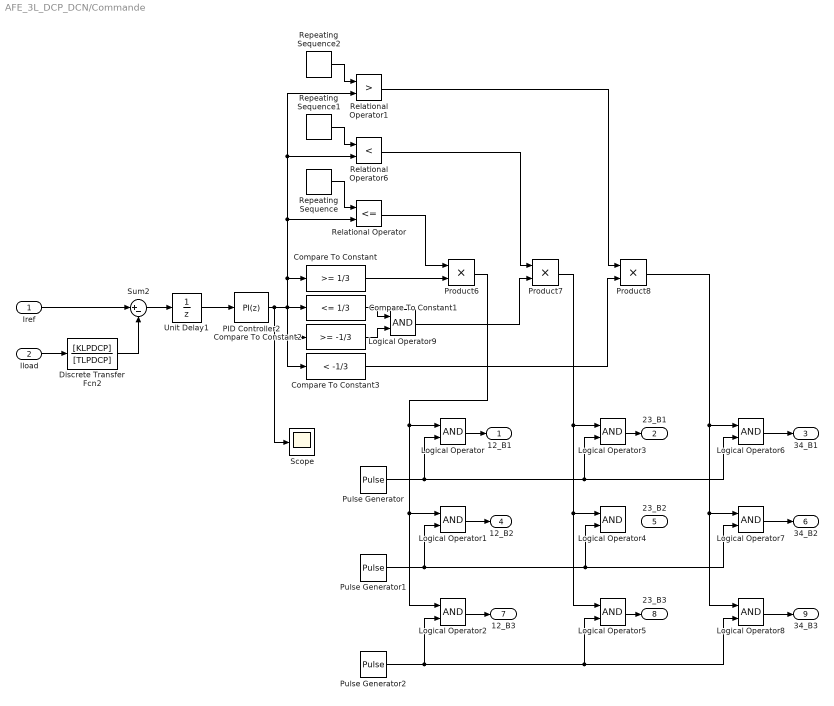
== system AFE_3L_DCP_DCN/Commande ==
  Iref : Inport
  "Iload " : Inport  Port=2
  Compare To Constant : simulink/Logic and Bit Operations/Compare To Constant  relop=>=  const=1/3  OutDataTypeStr=boolean
  Compare To Constant1 : simulink/Logic and Bit Operations/Compare To Constant  relop=<=  const=1/3  OutDataTypeStr=boolean
  Compare To Constant2 : simulink/Logic and Bit Operations/Compare To Constant  relop=>=  const=-1/3  OutDataTypeStr=boolean
  Compare To Constant3 : simulink/Logic and Bit Operations/Compare To Constant  relop=<  const=-1/3  OutDataTypeStr=boolean
  Discrete Transfer Fcn2 : DiscreteTransferFcn  Numerator=[KLPDCP]  Denominator=[TLPDCP]  SampleTime=Tpas
  Logical Operator{,1..9} (10 alike) : Logic  AllPortsSameDT=off  OutDataTypeStr=boolean  SampleTime=Tpas
  PID Controller2 : simulink/Continuous/PID Controller  Controller=PI  TimeDomain=Discrete-time  SampleTime=Tpas  IntegratorMethod=Forward Euler  FilterMethod=Forward Euler  Form=Parallel  P=PDCP  I=IDCP  D=0  N=100  InitialConditionSource=internal  InitialConditionForIntegrator=0  InitialConditionForFilter=0  ExternalReset=none  LimitOutput=on  UpperSaturationLimit=1  LowerSaturationLimit=-1  LinearizeAsGain=on  AntiWindupMode=clamping  Kb=1  TrackingMode=off  Kt=1  PParamMin=[]  PParamMax=[]  IParamMin=[]  IParamMax=[]  DParamMin=[]  DParamMax=[]  NParamMin=[]  NParamMax=[]  KbParamMin=[]  KbParamMax=[]  KtParamMin=[]  KtParamMax=[]  POutMin=[]  POutMax=[]  IOutMin=[]  IOutMax=[]  DOutMin=[]  DOutMax=[]  NOutMin=[]  NOutMax=[]  KbOutMin=[]  KbOutMax=[]  KtOutMin=[]  KtOutMax=[]  IntegratorOutMin=[]  IntegratorOutMax=[]  FilterOutMin=[]  FilterOutMax=[]  SumOutMin=[]  SumOutMax=[]  SumI1OutMin=[]  SumI1OutMax=[]  SumI2OutMin=[]  SumI2OutMax=[]  SumI3OutMin=[]  SumI3OutMax=[]  SumDOutMin=[]  SumDOutMax=[]  SaturationOutMin=[]  SaturationOutMax=[]  IntegratorContinuousStateAttributes=''  IntegratorStateMustResolveToSignalObject=off  IntegratorRTWStateStorageClass=Auto  FilterContinuousStateAttributes=''  FilterStateMustResolveToSignalObject=off  FilterRTWStateStorageClass=Auto
  Product6 : Product  SampleTime=Tpas
  Product7 : Product  SampleTime=Tpas
  Product8 : Product  SampleTime=Tpas
  Pulse Generator : DiscretePulseGenerator  Period=floor(1/(fmod4Q/3) * 1/Tpas)  PulseWidth=floor(1/(fmod4Q) * 1/Tpas)  SampleTime=Tpas
  Pulse Generator1 : DiscretePulseGenerator  Period=floor(1/(fmod4Q/3) * 1/Tpas)  PulseWidth=floor(1/(fmod4Q) * 1/Tpas)  PhaseDelay=floor(1/(fmod4Q) * 1/Tpas)  SampleTime=Tpas
  Pulse Generator2 : DiscretePulseGenerator  Period=floor(1/(fmod4Q/3) * 1/Tpas)  PulseWidth=floor(1/(fmod4Q) * 1/Tpas)  PhaseDelay=floor(2/(fmod4Q) * 1/Tpas)  SampleTime=Tpas
  Relational Operator : RelationalOperator  Operator=<=  OutDataTypeStr=boolean
  Relational Operator1 : RelationalOperator  Operator=>  OutDataTypeStr=boolean
  Relational Operator6 : RelationalOperator  Operator=<  OutDataTypeStr=boolean
  Repeating Sequence : simulink/Sources/Repeating Sequence  rep_seq_t=[0 1/fmod4Q]  rep_seq_y=[1/3 1.035]
  Repeating Sequence1 : simulink/Sources/Repeating Sequence  rep_seq_t=[0 1/fmod4Q]  rep_seq_y=[-.35 .35]
  Repeating Sequence2 : simulink/Sources/Repeating Sequence  rep_seq_t=[0 1/fmod4Q]  rep_seq_y=[-1 -1/3]
  Scope : Scope
      settings: SaveName=ScopeData3
  Sum2 : Sum  Inputs=|+-
  Unit Delay1 : UnitDelay  SampleTime=-1
  12_B1 : Outport
  23_B1 : Outport  Port=2
  34_B1 : Outport  Port=3
  12_B2 : Outport  Port=4
  23_B2 : Outport  Port=5
  34_B2 : Outport  Port=6
  12_B3 : Outport  Port=7
  23_B3 : Outport  Port=8
  34_B3 : Outport  Port=9
  wires:
  Compare To Constant/1 -> Product6/2
  Compare To Constant3/1 -> Product8/2
  Compare To Constant1/1 -> Logical Operator9/1
  Compare To Constant2/1 -> Logical Operator9/2
  Logical Operator9/1 -> Product7/2
  Repeating Sequence/1 -> Relational Operator/1
  Repeating Sequence2/1 -> Relational Operator1/1
  Relational Operator/1 -> Product6/1
  Relational Operator6/1 -> Product7/1
  Relational Operator1/1 -> Product8/1
  PID Controller2/1 -> Scope/1, Relational Operator/2, Relational Operator1/2, Relational Operator6/2, Compare To Constant/1, Compare To Constant1/1, Compare To Constant3/1, Compare To Constant2/1
  Repeating Sequence1/1 -> Relational Operator6/1
  Iref/1 -> Sum2/1
  "Iload "/1 -> Discrete Transfer Fcn2/1
  Discrete Transfer Fcn2/1 -> Sum2/2
  Sum2/1 -> Unit Delay1/1
  Unit Delay1/1 -> PID Controller2/1
  Product6/1 -> Logical Operator2/1, Logical Operator1/1, Logical Operator/1
  Pulse Generator2/1 -> Logical Operator5/2, Logical Operator8/2, Logical Operator2/2
  Pulse Generator/1 -> Logical Operator3/2, Logical Operator6/2, Logical Operator/2
  Pulse Generator1/1 -> Logical Operator1/2, Logical Operator4/2, Logical Operator7/2
  Product7/1 -> Logical Operator5/1, Logical Operator4/1, Logical Operator3/1
  Product8/1 -> Logical Operator8/1, Logical Operator7/1, Logical Operator6/1
  Logical Operator/1 -> 12_B1/1
  Logical Operator8/1 -> 34_B3/1
  Logical Operator1/1 -> 12_B2/1
  Logical Operator3/1 -> 23_B1/1
  Logical Operator6/1 -> 34_B1/1
  Logical Operator2/1 -> 12_B3/1
  Logical Operator5/1 -> 23_B3/1
  Logical Operator7/1 -> 34_B2/1

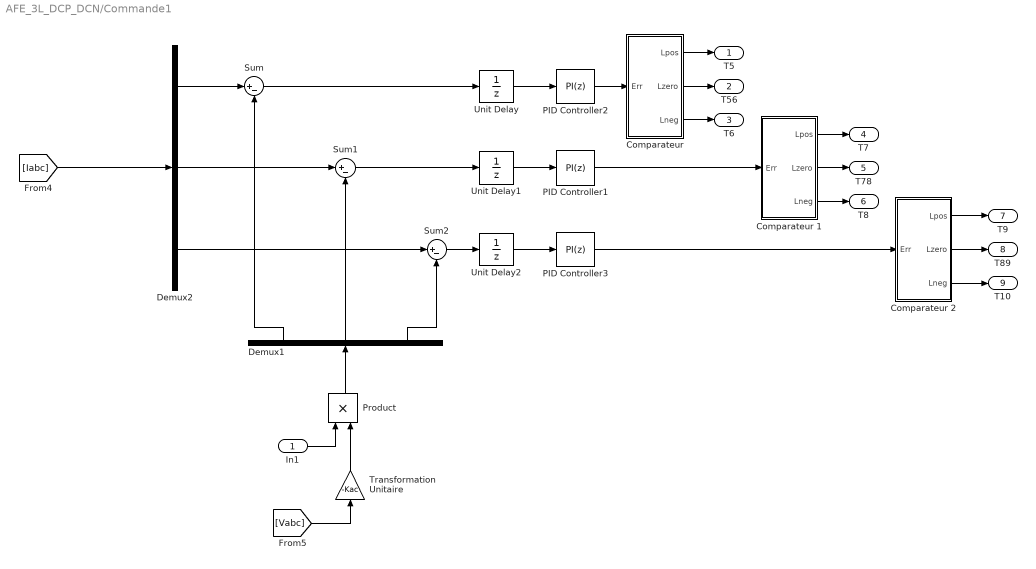
== system AFE_3L_DCP_DCN/Commande1 ==
  In1 : Inport
  "Comparateur " : Subsystem
  Comparateur 1 : Subsystem
  Comparateur 2 : Subsystem
  Demux1 : Demux  Outputs=3
  Demux2 : Demux  Outputs=3
  PID Controller1 : simulink/Continuous/PID Controller  Controller=PI  TimeDomain=Discrete-time  SampleTime=Tpas  IntegratorMethod=Forward Euler  FilterMethod=Forward Euler  Form=Parallel  P=PC  I=IC  D=0  N=100  InitialConditionSource=internal  InitialConditionForIntegrator=0  InitialConditionForFilter=0  ExternalReset=none  LimitOutput=on  UpperSaturationLimit=0.95  LowerSaturationLimit=-0.95  LinearizeAsGain=on  AntiWindupMode=clamping  Kb=1  TrackingMode=off  Kt=1  PParamMin=[]  PParamMax=[]  IParamMin=[]  IParamMax=[]  DParamMin=[]  DParamMax=[]  NParamMin=[]  NParamMax=[]  KbParamMin=[]  KbParamMax=[]  KtParamMin=[]  KtParamMax=[]  POutMin=[]  POutMax=[]  IOutMin=[]  IOutMax=[]  DOutMin=[]  DOutMax=[]  NOutMin=[]  NOutMax=[]  KbOutMin=[]  KbOutMax=[]  KtOutMin=[]  KtOutMax=[]  IntegratorOutMin=[]  IntegratorOutMax=[]  FilterOutMin=[]  FilterOutMax=[]  SumOutMin=[]  SumOutMax=[]  SumI1OutMin=[]  SumI1OutMax=[]  SumI2OutMin=[]  SumI2OutMax=[]  SumI3OutMin=[]  SumI3OutMax=[]  SumDOutMin=[]  SumDOutMax=[]  SaturationOutMin=[]  SaturationOutMax=[]  IntegratorContinuousStateAttributes=''  IntegratorStateMustResolveToSignalObject=off  IntegratorRTWStateStorageClass=Auto  FilterContinuousStateAttributes=''  FilterStateMustResolveToSignalObject=off  FilterRTWStateStorageClass=Auto
  PID Controller2 : simulink/Continuous/PID Controller  Controller=PI  TimeDomain=Discrete-time  SampleTime=Tpas  IntegratorMethod=Forward Euler  FilterMethod=Forward Euler  Form=Parallel  P=PC  I=IC  D=0  N=100  InitialConditionSource=internal  InitialConditionForIntegrator=0  InitialConditionForFilter=0  ExternalReset=none  LimitOutput=on  UpperSaturationLimit=0.95  LowerSaturationLimit=-0.95  LinearizeAsGain=on  AntiWindupMode=clamping  Kb=1  TrackingMode=off  Kt=1  PParamMin=[]  PParamMax=[]  IParamMin=[]  IParamMax=[]  DParamMin=[]  DParamMax=[]  NParamMin=[]  NParamMax=[]  KbParamMin=[]  KbParamMax=[]  KtParamMin=[]  KtParamMax=[]  POutMin=[]  POutMax=[]  IOutMin=[]  IOutMax=[]  DOutMin=[]  DOutMax=[]  NOutMin=[]  NOutMax=[]  KbOutMin=[]  KbOutMax=[]  KtOutMin=[]  KtOutMax=[]  IntegratorOutMin=[]  IntegratorOutMax=[]  FilterOutMin=[]  FilterOutMax=[]  SumOutMin=[]  SumOutMax=[]  SumI1OutMin=[]  SumI1OutMax=[]  SumI2OutMin=[]  SumI2OutMax=[]  SumI3OutMin=[]  SumI3OutMax=[]  SumDOutMin=[]  SumDOutMax=[]  SaturationOutMin=[]  SaturationOutMax=[]  IntegratorContinuousStateAttributes=''  IntegratorStateMustResolveToSignalObject=off  IntegratorRTWStateStorageClass=Auto  FilterContinuousStateAttributes=''  FilterStateMustResolveToSignalObject=off  FilterRTWStateStorageClass=Auto
  PID Controller3 : simulink/Continuous/PID Controller  Controller=PI  TimeDomain=Discrete-time  SampleTime=Tpas  IntegratorMethod=Forward Euler  FilterMethod=Forward Euler  Form=Parallel  P=PC  I=IC  D=0  N=100  InitialConditionSource=internal  InitialConditionForIntegrator=0  InitialConditionForFilter=0  ExternalReset=none  LimitOutput=on  UpperSaturationLimit=0.95  LowerSaturationLimit=-0.95  LinearizeAsGain=on  AntiWindupMode=clamping  Kb=1  TrackingMode=off  Kt=1  PParamMin=[]  PParamMax=[]  IParamMin=[]  IParamMax=[]  DParamMin=[]  DParamMax=[]  NParamMin=[]  NParamMax=[]  KbParamMin=[]  KbParamMax=[]  KtParamMin=[]  KtParamMax=[]  POutMin=[]  POutMax=[]  IOutMin=[]  IOutMax=[]  DOutMin=[]  DOutMax=[]  NOutMin=[]  NOutMax=[]  KbOutMin=[]  KbOutMax=[]  KtOutMin=[]  KtOutMax=[]  IntegratorOutMin=[]  IntegratorOutMax=[]  FilterOutMin=[]  FilterOutMax=[]  SumOutMin=[]  SumOutMax=[]  SumI1OutMin=[]  SumI1OutMax=[]  SumI2OutMin=[]  SumI2OutMax=[]  SumI3OutMin=[]  SumI3OutMax=[]  SumDOutMin=[]  SumDOutMax=[]  SaturationOutMin=[]  SaturationOutMax=[]  IntegratorContinuousStateAttributes=''  IntegratorStateMustResolveToSignalObject=off  IntegratorRTWStateStorageClass=Auto  FilterContinuousStateAttributes=''  FilterStateMustResolveToSignalObject=off  FilterRTWStateStorageClass=Auto
  Product : Product
  Sum : Sum  Inputs=|+-
  Sum1 : Sum  Inputs=|+-
  Sum2 : Sum  Inputs=|+-
  Transformation Unitaire : Gain  Gain=-Kac
  Unit Delay : UnitDelay  SampleTime=-1
  Unit Delay1 : UnitDelay  SampleTime=-1
  Unit Delay2 : UnitDelay  SampleTime=-1
  T5 : Outport
  T56 : Outport  Port=2
  T6 : Outport  Port=3
  T7 : Outport  Port=4
  T78 : Outport  Port=5
  T8 : Outport  Port=6
  T9 : Outport  Port=7
  T89 : Outport  Port=8
  T10 : Outport  Port=9
  wires:
  Demux2/1 -> Sum/1
  Demux2/2 -> Sum1/1
  Demux2/3 -> Sum2/1
  Sum/1 -> Unit Delay/1
  Sum1/1 -> Unit Delay1/1
  Sum2/1 -> Unit Delay2/1
  Unit Delay/1 -> PID Controller2/1
  Unit Delay1/1 -> PID Controller1/1
  Unit Delay2/1 -> PID Controller3/1
  [Iabc] -> Demux2/1
  [Vabc] -> Transformation Unitaire/1
  Demux1/1 -> Sum/2
  Demux1/2 -> Sum1/2
  Demux1/3 -> Sum2/2
  Transformation Unitaire/1 -> Product/2
  In1/1 -> Product/1
  Product/1 -> Demux1/1
  PID Controller2/1 -> "Comparateur "/1(Err)
  PID Controller1/1 -> Comparateur 1/1(Err)
  PID Controller3/1 -> Comparateur 2/1(Err)
  "Comparateur "/1(Lpos) -> T5/1
  "Comparateur "/3(Lneg) -> T6/1
  "Comparateur "/2(Lzero) -> T56/1
  Comparateur 1/1(Lpos) -> T7/1
  Comparateur 1/3(Lneg) -> T8/1
  Comparateur 1/2(Lzero) -> T78/1
  Comparateur 2/1(Lpos) -> T9/1
  Comparateur 2/3(Lneg) -> T10/1
  Comparateur 2/2(Lzero) -> T89/1

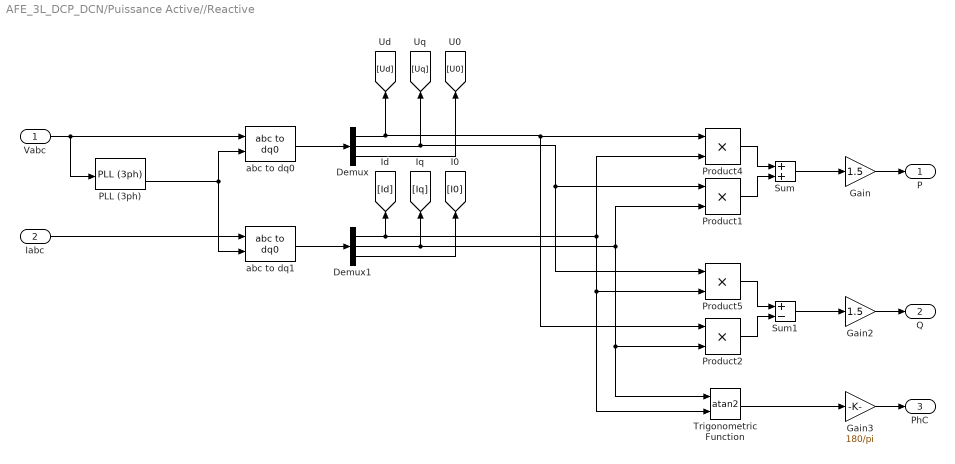
== system AFE_3L_DCP_DCN/Puissance Active//Reactive ==
  Vabc : Inport
  Iabc : Inport  Port=2
  Demux : Demux  Outputs=3
  Demux1 : Demux  Outputs=3
  Gain : Gain  Gain=1.5
  Gain2 : Gain  Gain=1.5
  Gain3 : Gain  Gain=180/pi
  PLL (3ph) : powerlib_meascontrol/PLL/PLL (3ph)  Fmin=49  Par_Init=[0, 50]  ParK=[180, 3200, 1]  TcD=1e-4  MaxRateChangeFreq=6  FilterCutOffFreq=25  Ts=Tpas  AGC=on
  Product{1..2,4..5} (4 alike) : Product
  Sum : Sum
  Sum1 : Sum  Inputs=+-
  Trigonometric Function : Trigonometry  Operator=atan2
  abc to dq0 : powerlib_meascontrol/Transformations/abc to dq0  Alignment=90 degrees behind phase A axis
  abc to dq1 : powerlib_meascontrol/Transformations/abc to dq0  Alignment=90 degrees behind phase A axis
  P : Outport
  Q : Outport  Port=2
  PhC : Outport  Port=3
  wires:
  Vabc/1 -> PLL (3ph)/1, abc to dq0/1
  abc to dq0/1 -> Demux/1
  abc to dq1/1 -> Demux1/1
  Product2/1 -> Sum1/2
  Sum1/1 -> Gain2/1
  Demux/3 -> [U0]
  Demux/2 -> Product5/1, Product1/1, [Uq]
  Demux/1 -> Product2/1, Product4/1, [Ud]
  Demux1/2 -> [Iq], Trigonometric Function/1, Product2/2, Product1/2
  Product5/1 -> Sum1/1
  Gain2/1 -> Q/1
  Trigonometric Function/1 -> Gain3/1
  Gain3/1 -> PhC/1
  Product4/1 -> Sum/1
  Product1/1 -> Sum/2
  Sum/1 -> Gain/1
  Gain/1 -> P/1
  Demux1/1 -> [Id], Trigonometric Function/2, Product5/2, Product4/2
  Demux1/3 -> [I0]
  PLL (3ph)/2 -> abc to dq1/2, abc to dq0/2
  Iabc/1 -> abc to dq1/1

== system AFE_3L_DCP_DCN/Subsystem ==

== system AFE_3L_DCP_DCN/Subsystem1 ==

== system AFE_3L_DCP_DCN/Subsystem2 ==

== system AFE_3L_DCP_DCN/Subsystem3 ==

== system AFE_3L_DCP_DCN/Subsystem4 ==

== system AFE_3L_DCP_DCN/Subsystem5 ==

== system AFE_3L_DCP_DCN/Subsystem6 ==

== system AFE_3L_DCP_DCN/Subsystem7 ==

== system AFE_3L_DCP_DCN/Subsystem8 ==

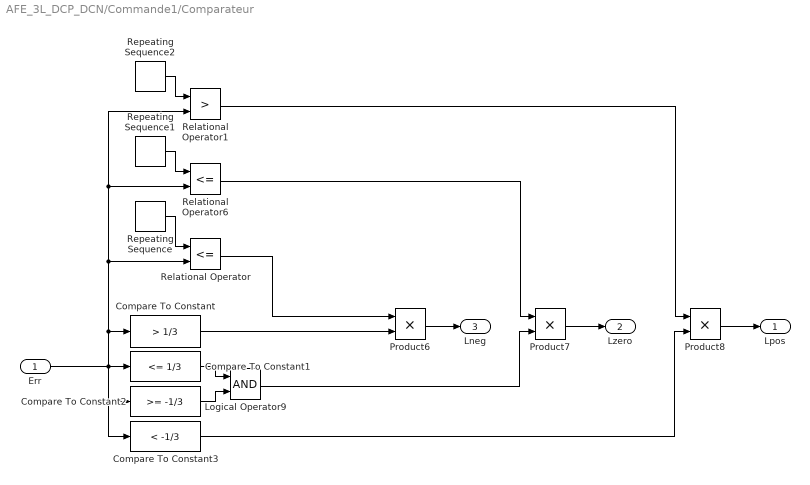
== system AFE_3L_DCP_DCN/Commande1/Comparateur  ==
  Err : Inport
  Compare To Constant : simulink/Logic and Bit Operations/Compare To Constant  relop=>  const=1/3  OutDataTypeStr=boolean
  Compare To Constant1 : simulink/Logic and Bit Operations/Compare To Constant  relop=<=  const=1/3  OutDataTypeStr=boolean
  Compare To Constant2 : simulink/Logic and Bit Operations/Compare To Constant  relop=>=  const=-1/3  OutDataTypeStr=boolean
  Compare To Constant3 : simulink/Logic and Bit Operations/Compare To Constant  relop=<  const=-1/3  OutDataTypeStr=boolean
  Logical Operator9 : Logic  AllPortsSameDT=off  OutDataTypeStr=boolean  SampleTime=Tpas
  Product6 : Product  SampleTime=Tpas
  Product7 : Product  SampleTime=Tpas
  Product8 : Product  SampleTime=Tpas
  Relational Operator : RelationalOperator  Operator=<=  OutDataTypeStr=boolean
  Relational Operator1 : RelationalOperator  Operator=>  OutDataTypeStr=boolean
  Relational Operator6 : RelationalOperator  Operator=<=  OutDataTypeStr=boolean
  Repeating Sequence : simulink/Sources/Repeating Sequence  rep_seq_t=[0 1e-3]  rep_seq_y=[1/3 1.035]
  Repeating Sequence1 : simulink/Sources/Repeating Sequence  rep_seq_t=[0 1e-3]  rep_seq_y=[-.35 .35]
  Repeating Sequence2 : simulink/Sources/Repeating Sequence  rep_seq_t=[0 1e-3]  rep_seq_y=[-1 -1/3]
  Lpos : Outport
  Lzero : Outport  Port=2
  Lneg : Outport  Port=3
  wires:
  Compare To Constant/1 -> Product6/2
  Compare To Constant3/1 -> Product8/2
  Compare To Constant1/1 -> Logical Operator9/1
  Compare To Constant2/1 -> Logical Operator9/2
  Logical Operator9/1 -> Product7/2
  Repeating Sequence/1 -> Relational Operator/1
  Repeating Sequence2/1 -> Relational Operator1/1
  Relational Operator/1 -> Product6/1
  Relational Operator6/1 -> Product7/1
  Relational Operator1/1 -> Product8/1
  Product6/1 -> Lneg/1
  Product8/1 -> Lpos/1
  Product7/1 -> Lzero/1
  Err/1 -> Relational Operator/2, Relational Operator1/2, Relational Operator6/2, Compare To Constant/1, Compare To Constant1/1, Compare To Constant3/1, Compare To Constant2/1
  Repeating Sequence1/1 -> Relational Operator6/1

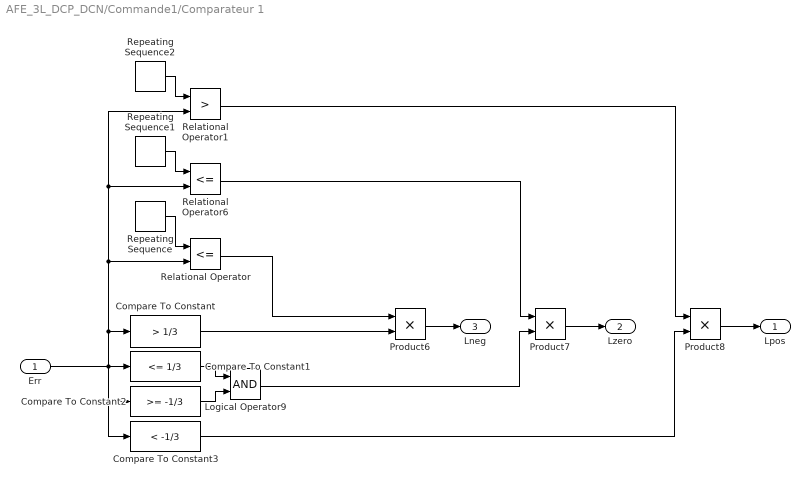
== system AFE_3L_DCP_DCN/Commande1/Comparateur 1 ==
  Err : Inport
  Compare To Constant : simulink/Logic and Bit Operations/Compare To Constant  relop=>  const=1/3  OutDataTypeStr=boolean
  Compare To Constant1 : simulink/Logic and Bit Operations/Compare To Constant  relop=<=  const=1/3  OutDataTypeStr=boolean
  Compare To Constant2 : simulink/Logic and Bit Operations/Compare To Constant  relop=>=  const=-1/3  OutDataTypeStr=boolean
  Compare To Constant3 : simulink/Logic and Bit Operations/Compare To Constant  relop=<  const=-1/3  OutDataTypeStr=boolean
  Logical Operator9 : Logic  AllPortsSameDT=off  OutDataTypeStr=boolean  SampleTime=Tpas
  Product6 : Product  SampleTime=Tpas
  Product7 : Product  SampleTime=Tpas
  Product8 : Product  SampleTime=Tpas
  Relational Operator : RelationalOperator  Operator=<=  OutDataTypeStr=boolean
  Relational Operator1 : RelationalOperator  Operator=>  OutDataTypeStr=boolean
  Relational Operator6 : RelationalOperator  Operator=<=  OutDataTypeStr=boolean
  Repeating Sequence : simulink/Sources/Repeating Sequence  rep_seq_t=[0 1e-3]  rep_seq_y=[1/3 1.035]
  Repeating Sequence1 : simulink/Sources/Repeating Sequence  rep_seq_t=[0 1e-3]  rep_seq_y=[-.35 .35]
  Repeating Sequence2 : simulink/Sources/Repeating Sequence  rep_seq_t=[0 1e-3]  rep_seq_y=[-1 -1/3]
  Lpos : Outport
  Lzero : Outport  Port=2
  Lneg : Outport  Port=3
  wires:
  Compare To Constant/1 -> Product6/2
  Compare To Constant3/1 -> Product8/2
  Compare To Constant1/1 -> Logical Operator9/1
  Compare To Constant2/1 -> Logical Operator9/2
  Logical Operator9/1 -> Product7/2
  Repeating Sequence/1 -> Relational Operator/1
  Repeating Sequence2/1 -> Relational Operator1/1
  Relational Operator/1 -> Product6/1
  Relational Operator6/1 -> Product7/1
  Relational Operator1/1 -> Product8/1
  Product6/1 -> Lneg/1
  Product8/1 -> Lpos/1
  Product7/1 -> Lzero/1
  Err/1 -> Relational Operator/2, Relational Operator1/2, Relational Operator6/2, Compare To Constant/1, Compare To Constant1/1, Compare To Constant3/1, Compare To Constant2/1
  Repeating Sequence1/1 -> Relational Operator6/1

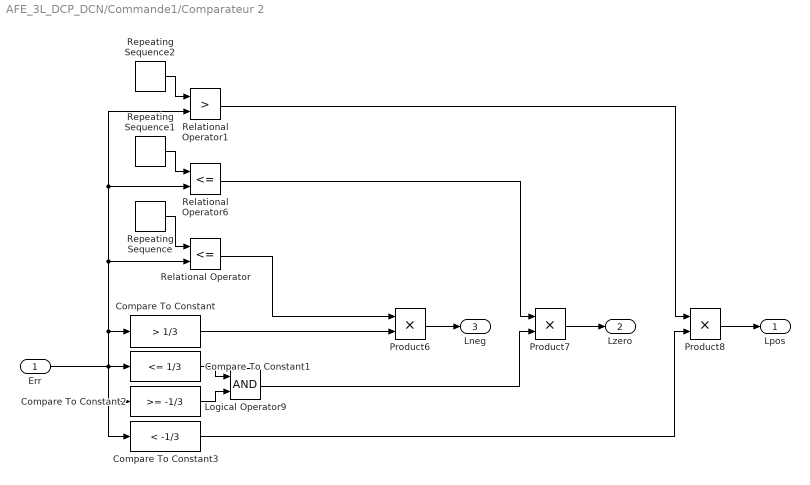
== system AFE_3L_DCP_DCN/Commande1/Comparateur 2 ==
  Err : Inport
  Compare To Constant : simulink/Logic and Bit Operations/Compare To Constant  relop=>  const=1/3  OutDataTypeStr=boolean
  Compare To Constant1 : simulink/Logic and Bit Operations/Compare To Constant  relop=<=  const=1/3  OutDataTypeStr=boolean
  Compare To Constant2 : simulink/Logic and Bit Operations/Compare To Constant  relop=>=  const=-1/3  OutDataTypeStr=boolean
  Compare To Constant3 : simulink/Logic and Bit Operations/Compare To Constant  relop=<  const=-1/3  OutDataTypeStr=boolean
  Logical Operator9 : Logic  AllPortsSameDT=off  OutDataTypeStr=boolean  SampleTime=Tpas
  Product6 : Product  SampleTime=Tpas
  Product7 : Product  SampleTime=Tpas
  Product8 : Product  SampleTime=Tpas
  Relational Operator : RelationalOperator  Operator=<=  OutDataTypeStr=boolean
  Relational Operator1 : RelationalOperator  Operator=>  OutDataTypeStr=boolean
  Relational Operator6 : RelationalOperator  Operator=<=  OutDataTypeStr=boolean
  Repeating Sequence : simulink/Sources/Repeating Sequence  rep_seq_t=[0 1e-3]  rep_seq_y=[1/3 1.035]
  Repeating Sequence1 : simulink/Sources/Repeating Sequence  rep_seq_t=[0 1e-3]  rep_seq_y=[-.35 .35]
  Repeating Sequence2 : simulink/Sources/Repeating Sequence  rep_seq_t=[0 1e-3]  rep_seq_y=[-1 -1/3]
  Lpos : Outport
  Lzero : Outport  Port=2
  Lneg : Outport  Port=3
  wires:
  Compare To Constant/1 -> Product6/2
  Compare To Constant3/1 -> Product8/2
  Compare To Constant1/1 -> Logical Operator9/1
  Compare To Constant2/1 -> Logical Operator9/2
  Logical Operator9/1 -> Product7/2
  Repeating Sequence/1 -> Relational Operator/1
  Repeating Sequence2/1 -> Relational Operator1/1
  Relational Operator/1 -> Product6/1
  Relational Operator6/1 -> Product7/1
  Relational Operator1/1 -> Product8/1
  Product6/1 -> Lneg/1
  Product8/1 -> Lpos/1
  Product7/1 -> Lzero/1
  Err/1 -> Relational Operator/2, Relational Operator1/2, Relational Operator6/2, Compare To Constant/1, Compare To Constant1/1, Compare To Constant3/1, Compare To Constant2/1
  Repeating Sequence1/1 -> Relational Operator6/1
